simulink model "dubins"  (R2021a)
settings: Solver=VariableStepAuto  StartTime=0.0  StopTime=20  RelTol=1e-3
libraries: simulink x1
settings Model: Creator=jiaweichen  LastModifiedBy=jiaweichen

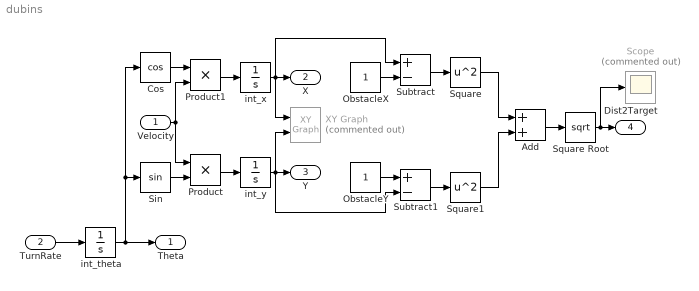
== system dubins ==
  Velocity : Inport
  TurnRate : Inport  Port=2
  Add : Sum
  Cos : Trigonometry  Operator=cos
  ObstacleX : Constant
  ObstacleY : Constant
  Product : Product
  Product1 : Product
  Scope : Scope  Commented=on
  Sin : Trigonometry
  Square : Math  Operator=square  SaturateOnIntegerOverflow=on
  Square Root : Sqrt  SaturateOnIntegerOverflow=on
  Square1 : Math  Operator=square  SaturateOnIntegerOverflow=on
  Subtract : Sum  Inputs=+-
  Subtract1 : Sum  Inputs=+-
  XY Graph : simulink/Sinks/XY Graph  Commented=on  xmin=-1  xmax=1  ymin=-1  ymax=1  st=-1
  int_theta : Integrator
  int_x : Integrator
  int_y : Integrator
  Theta : Outport
  X : Outport  Port=2
  Y : Outport  Port=3
  Dist2Target : Outport  Port=4
  wires:
  TurnRate/1 -> int_theta/1
  int_theta/1 -> Cos/1, Sin/1, Theta/1
  Sin/1 -> Product/2
  Velocity/1 -> Product/1, Product1/2
  Cos/1 -> Product1/1
  Product1/1 -> int_x/1
  Product/1 -> int_y/1
  int_x/1 -> Subtract/1, XY Graph/1, X/1
  int_y/1 -> XY Graph/2, Subtract1/2, Y/1
  ObstacleX/1 -> Subtract/2
  ObstacleY/1 -> Subtract1/1
  Subtract/1 -> Square/1
  Subtract1/1 -> Square1/1
  Square/1 -> Add/1
  Square1/1 -> Add/2
  Add/1 -> Square Root/1
  Square Root/1 -> Scope/1, Dist2Target/1
